simulink library "calcDistanceFromPath"  (R2020a)
settings: Solver=VariableStepAuto  StartTime=0.0  StopTime=10.0  RelTol=1e-3
libraries: calculate_vector_magnitude x1, calc_path_coordinates x1
settings Model: Creator=Ayaz  LastModifiedBy=Ayaz

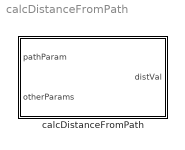
== system calcDistanceFromPath ==
  calcDistanceFromPath : Subsystem

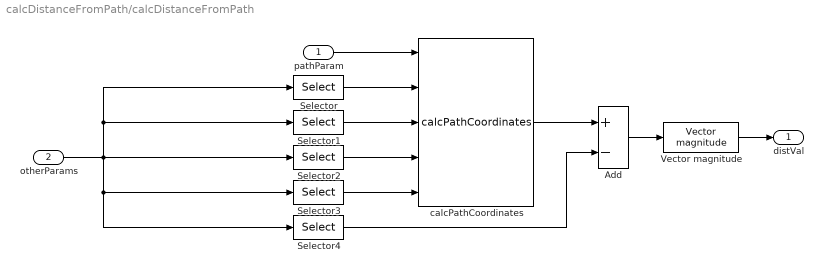
== system calcDistanceFromPath/calcDistanceFromPath ==
  pathParam : Inport
  otherParams : Inport  Port=2
  Add : Sum  Inputs=+-
  Selector : Selector  InputPortWidth=8  IndexOptions=Index vector (dialog)  Indices=1  OutputSizes=1
  Selector1 : Selector  InputPortWidth=8  IndexOptions=Index vector (dialog)  Indices=2  OutputSizes=1
  Selector2 : Selector  InputPortWidth=8  IndexOptions=Index vector (dialog)  Indices=3  OutputSizes=1
  Selector3 : Selector  InputPortWidth=8  IndexOptions=Index vector (dialog)  Indices=4  OutputSizes=1
  Selector4 : Selector  InputPortWidth=8  IndexOptions=Index vector (dialog)  Indices=[5 6 7]  OutputSizes=1
  Vector magnitude : calculate_vector_magnitude/Vector magnitude  SystemSampleTime=-1  Latency=0  AutoFrameSizeCalculation=off
  calcPathCoordinates : calc_path_coordinates/calcPathCoordinates  SystemSampleTime=-1  Latency=0  AutoFrameSizeCalculation=off
  distVal : Outport
  wires:
  Vector magnitude/1 -> distVal/1
  otherParams/1 -> Selector4/1, Selector3/1, Selector/1, Selector1/1, Selector2/1
  pathParam/1 -> calcPathCoordinates/1
  Selector/1 -> calcPathCoordinates/2
  Selector1/1 -> calcPathCoordinates/3
  Selector2/1 -> calcPathCoordinates/4
  Selector3/1 -> calcPathCoordinates/5
  calcPathCoordinates/1 -> Add/1
  Selector4/1 -> Add/2
  Add/1 -> Vector magnitude/1
